simulink model "ESC_sails"  (R2020b)
settings: Solver=VariableStepAuto  StartTime=0.0  StopTime=100  RelTol=1e-3
libraries: simulink_extras x1
settings Model: Creator=Calle  LastModifiedBy=Calle

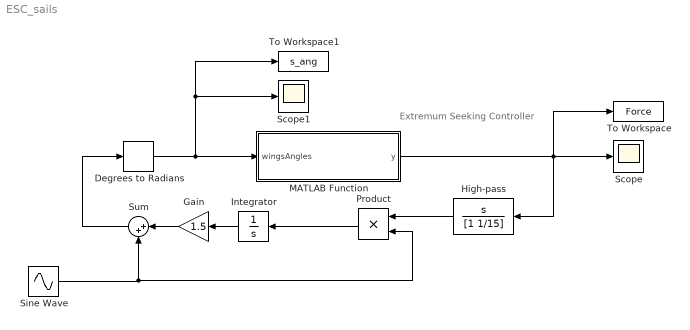
== system ESC_sails ==
  note: Extremum Seeking Controller
  Degrees to Radians : simulink_extras/Transformations/Degrees to Radians
  Gain : Gain  Gain=1.5
  High-pass : TransferFcn  Numerator=[1 0]  Denominator=[1 1/15]
  Integrator : Integrator
  MATLAB Function : MATLAB Function  TreatAsAtomicUnit=on
  Product : Product
  Scope : Scope
  Scope1 : Scope
  Sine Wave : Sin  Frequency=1/10*2*pi  SampleTime=0
  Sum : Sum  Inputs=|++
  To Workspace : ToWorkspace  VariableName=Force  SaveFormat=Timeseries  SampleTime=-1
  To Workspace1 : ToWorkspace  VariableName=s_ang  SaveFormat=Timeseries  SampleTime=-1
  wires:
  Degrees to Radians/1 -> To Workspace1/1, Scope1/1, MATLAB Function/1(wingsAngles)
  High-pass/1 -> Product/1
  Integrator/1 -> Gain/1
  MATLAB Function/1(y) -> Scope/1, High-pass/1, To Workspace/1
  Sine Wave/1 -> Product/2, Sum/2
  Sum/1 -> Degrees to Radians/1
  Product/1 -> Integrator/1
  Gain/1 -> Sum/1

== matlab function ESC_sails/MATLAB Function ==
  data: wingsAngles input; y output
function y = fcn(wingsAngles)

addpath('code');

%% 2D trim angles from J

AWAvec = 45;%20:2.5:170;

flapsAngles = zeros(length(AWAvec),4);

%% Constant VLM parameters

% Environmental varibles
environment.tws 	= 10;   % Here used as freestream velocity, freestream is uniform
environment.rho 	= 1.2; % Air density
environment.vs  	= 0;   % not used
environment.mir     = 1;   % =1 for mirroring geometry in z = 0 in calculations. 

% Environmental varibles
global tws twa rho vs
tws = environment.tws; % Here used as freestream velocity, freestream is uniform
% twa = environment.twa; % True wind angle
rho = environment.rho; % Air density
vs  = environment.vs;  % not used
mir = environment.mir;

environment.inflow = 'uniform'; % can be: "BL", "twisted" or "uniform". BL: ITTC wind profile used, but no boat speed. Twisted: BL + boat speed accounted for
environment.zRef = 10; %m, height at which wind is defined
environment.windOffset = 29; % Offset from deck height (wing geomtrically close to 0hiehgt for miroring)
environment.BoatSpeed = 0*1852/3600; %Boat speed in m/s
environment.BoatKG = [100,0,25]; %From SSPA hydro in VPP

heelAngle = 0; 

dxW = 0.1925;                % Same for all wings in this case
flapPos= [-0.1148 ; 0 ;0 ];%[-6.7146; 0;0];    %  %Same for all wings in this case
dxF=0;                      % Same for all wings in this case

% RIGS DISRETIZATION
Nxwing = 3;                  % Same for all wings in this case
Nxflap = 6;                % Same for all flaps in this case
Nzall = 9;                 % Same for all flaps and wings, in all cases

% WAKE Parameters
wakeTypeAll = 'fixed'; 
wakeLengthAll = 100;
rCoreTot = 1e-10;
NxwakeWing = 1;
wakeCoreKr = 0.5; %kr Used only for wakeType free
wakeStepAll = 1; % Used only for wakeType free

% RIGS Postion and angles
originWing1 = [0.9; 0; 0];%[170; 0; 36];% 
originWing2 = [2.5; 0; 0];
originWing3 = [4.1; 0; 0];
originWing4 = [5.7; 0; 0];
originWings = [originWing1, originWing2, originWing3, originWing4];
%%

FA = zeros(length(AWAvec),2);
CEA = zeros(length(AWAvec),3);
Faero = zeros(length(AWAvec),2);
Maero = zeros(length(AWAvec),2);

for k = 1:length(AWAvec)
    clearvars rigs results
    
    geom = getGeometry('geom_7m_3.txt',dxW,flapPos,dxF);

    for ii = 1:4
        % ii=1;
        rigs(ii).wing = geom.wing;
        rigs(ii).wing.Nx = Nxwing;
        rigs(ii).wing.Nz = Nzall;
        rigs(ii).wing.Type = 'wing';
%       rigs(ii).wing.sheetAngle = deg2rad(wingAngle1);
        rigs(ii).wing.flapAngle = 0 ;        % Only uselful for flap but needed to have same struct
        rigs(ii).wing.flapAxis = [0; 0; 0];  % Only uselful for flap but needed to have same struct
        rigs(ii).wing.dX = dxW;
%       rigs(ii).wing.heelAngle = deg2rad(heelAngle);
        rigs(ii).wing.wingOrigin = originWings(:,ii);
        rigs(ii).wing.mir = mir;               % TO DO make mirorring with deck height
    
        rigs(ii).flap = geom.flap;
        rigs(ii).flap.Nx = Nxflap;
        rigs(ii).flap.Nz = Nzall;
        rigs(ii).flap.Type =  'flap';
%       rigs(ii).flap.sheetAngle = rigs(ii).wing.sheetAngle;
%       rigs(ii).flap.flapAngle = deg2rad(flapAngle1);
        rigs(ii).flap.flapAxis = flapPos;
        rigs(ii).flap.dX = dxF;
%       rigs(ii).flap.heelAngle = deg2rad(heelAngle);
        rigs(ii).flap.wingOrigin = originWings(:,ii);
        rigs(ii).flap.mir = mir;
%       rigs(ii).wing.panels = meshRig(rigs(ii).wing, 'linear');
%       rigs(ii).flap.panels = meshRig(rigs(ii).flap, 'linear');
    
        rigs(ii).Rcore = rCoreTot; % vortex core size
%       rigs(ii).panels = orderRigPanels(rigs(ii).wing,rigs(ii).flap);
        rigs(ii).Nx = rigs(ii).wing.Nx+rigs(ii).flap.Nx;
        rigs(ii).Nz = rigs(ii).wing.Nz;
        rigs(ii).mir = mir; % Used only to mirror the plots
        rigs(ii).wakeType = wakeTypeAll;
        rigs(ii).wakeLength = wakeLengthAll;
        rigs(ii).Nxw = NxwakeWing;
        rigs(ii).kr = wakeCoreKr;
        rigs(ii).wakeStep = wakeStepAll;
    end


    for ii = 1:length(rigs)
        rigs(ii).wing.sheetAngle = deg2rad(wingsAngles(k,ii));
        rigs(ii).wing.heelAngle = deg2rad(heelAngle);
        rigs(ii).flap.sheetAngle = rigs(ii).wing.sheetAngle;
        rigs(ii).flap.flapAngle = deg2rad(flapsAngles(k,ii));
        rigs(ii).flap.heelAngle = deg2rad(heelAngle);

        rigs(ii).wing.panels = meshRig(rigs(ii).wing, 'linear');
        rigs(ii).flap.panels = meshRig(rigs(ii).flap, 'linear');
        rigs(ii).panels = orderRigPanels(rigs(ii).wing,rigs(ii).flap);
    end


    twa = deg2rad(AWAvec(k));
    disp(AWAvec(k));

    rigs = preProcessor(rigs,environment);
    rigs = solver(rigs,mir,environment);
    if strcmp(wakeTypeAll,'free')
        rigs = freeWake(rigs,mir,environment);
        rigs = solver(rigs,mir,environment);
    end
    results = postProcessor(rigs, mir,environment);
%         if(k==1)
%            plotLattice(rigs,k);
%            plotPressure(rigs,results,k+100);
%            plotForces(rigs,results,k);
%         end
%        disp(sprintf('Lift: %.2f N',results(1).L));
%        disp(sprintf('Drag: %.2f N',results(1).D));

%         drawnow;
    FA(k,1) = results.CX;
    FA(k,2) = results.CY;
    FA(k,3) = results.CZ;

    Faero(k,1) = results.CL;
    Faero(k,2) = results.CD;

    CEA(k,1) = results.CEA;
    CEA(k,2) = results.CEY;
    CEA(k,3) = results.CEH;

    Maero(k,1)= (results(1).FY*((results(1).CEH+environment.windOffset)))/(0.5*1.2*tws^2*results(1).A);
    Maero(k,2)= (results(1).FX*(results(1).CEA-environment.BoatKG(1)))/(0.5*1.2*tws^2*results(1).A);
    Maero(k,3) = (results(1).FX*(results(1).CEY-environment.BoatKG(2))+...
    results(1).FY*(results(1).CEA-environment.BoatKG(1)))/(0.5*1.2*tws^2*results(1).A);

    
end

y = [results(1).fx,results(2).fx,results(3).fx,results(4).fx];
